simulink model "Teleoperation"  (R2020a)
settings: Solver=VariableStepAuto  StartTime=0.0  StopTime=inf  RelTol=1e-3
undefined symbols (not defined in the file or in its folder): currentCFG_Cognata_Amp_Tobi_split_UB, UB
libraries: robotlib x7, gtecHighspeedLib x2, TobiiEyeTrackerLib x1, gUSBamplib x1
settings Model: Creator=LAB-ORENMUZ  LastModifiedBy=LAB-OREN3
settings DataIOCC: ReturnWorkspaceOutputs=off
settings DebuggingCC: ArithmeticOperatorsInVariantConditions=warning
settings SFSimCC: SimUseLocalCustomCode=off  CustomCodeUndefinedFunction=UseInterfaceOnly
settings RTWCC: RTWUseLocalCustomCode=off
settings CodeAppCC: StateflowObjectComments=on

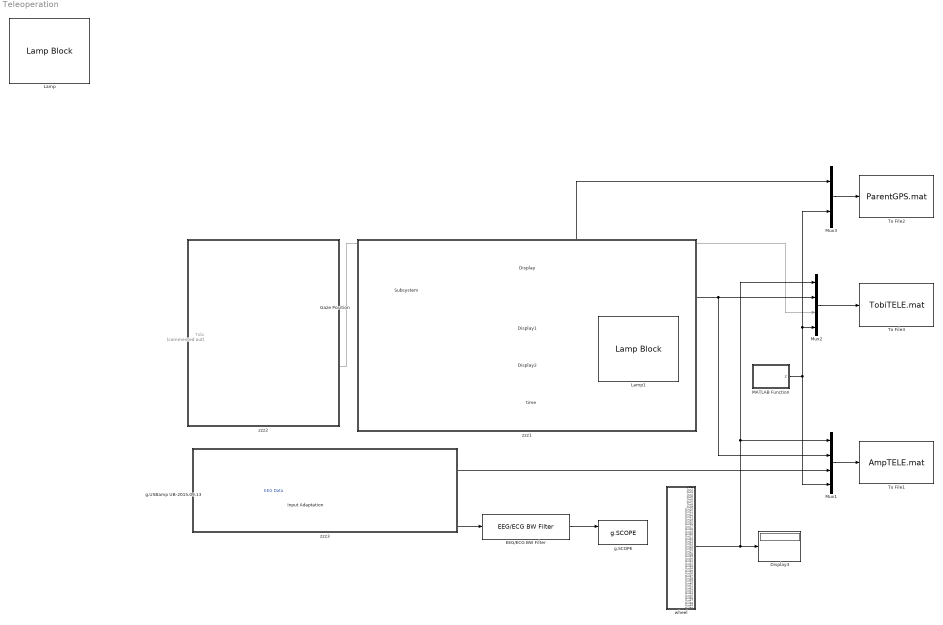
== system Teleoperation ==
  Display{,1..3} (4 alike) : Display
  EEG/ECG BW Filter : gtecHighspeedLib/EEG//ECG BW Filter  Order=6  LowerFreq=0.1  UpperFreq=30  SampFreq=512
      settings: SourceProductName=g.HIsys Library
  Gaze Position : Display
  Input Adaptation : Subsystem
  Lamp : LampBlock
  Lamp1 : LampBlock
  MATLAB Function : MATLAB Function  TreatAsAtomicUnit=on
  Mux1 : Mux
  Mux2 : Mux
  Mux3 : Mux  Inputs=2
  Subsystem : Subsystem
  To File1 : ToFile  Filename=AmpTELE.mat  MatrixName=AmpdataTELE
  To File2 : ToFile  Filename=ParentGPS.mat  MatrixName=Parent
  To File3 : ToFile  Filename=TobiTELE.mat  MatrixName=TobidataTELE
  Tobi : Subsystem  Commented=on
  g.SCOPE : gtecHighspeedLib/g.SCOPE
      settings: SourceProductName=g.HIsys Library
  g.USBamp UB-2015.09.13 : gUSBamplib/g.USBamp  cfg=currentCFG_Cognata_Amp_Tobi_split_UB-2015.09.13.cfg  snr=UB-2015.09.13
      settings: SourceProductName=g.USBamp
  time : Display
  wheel : Subsystem
  zzz1 : Subsystem  TreatAsAtomicUnit=on
      settings: OpenFcn=% no-op
      mask Display: disp('')
  zzz2 : Subsystem  TreatAsAtomicUnit=on
      settings: OpenFcn=% no-op
      mask Display: disp('')
  zzz3 : Subsystem  TreatAsAtomicUnit=on
      settings: OpenFcn=% no-op
      mask Display: disp('')
  wires:
  Subsystem/1(Out1) -> Display/1
  Subsystem/3(Out3) -> Display1/1
  Subsystem/4(Out4) -> Display2/1
  Tobi/2(Sum) -> Mux2/3
  Mux2/1 -> To File3/1
  EEG/ECG BW Filter/1 -> g.SCOPE/1
  Input Adaptation/1(Out) -> Mux1/3, EEG/ECG BW Filter/1
  Tobi/1(Gaze Pos) -> Gaze Position/1
  Subsystem/2(Out2) -> Mux1/2, Mux2/2, Mux3/1
  g.USBamp UB-2015.09.13/1 -> Input Adaptation/1(In)  "EEG Data"
  MATLAB Function/1(z) -> Mux1/4, Mux3/2, Mux2/4
  wheel/25(Out25) -> Mux2/1, Mux1/1, Display3/1
  Mux1/1 -> To File1/1
  Subsystem/5(Out5) -> time/1
  Mux3/1 -> To File2/1

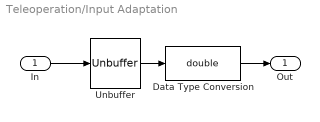
== system Teleoperation/Input Adaptation ==
  In : Inport
  Data Type Conversion : DataTypeConversion  OutDataTypeStr=double
  Unbuffer : Unbuffer
  Out : Outport
  wires:
  In/1 -> Unbuffer/1
  Unbuffer/1 -> Data Type Conversion/1
  Data Type Conversion/1 -> Out/1

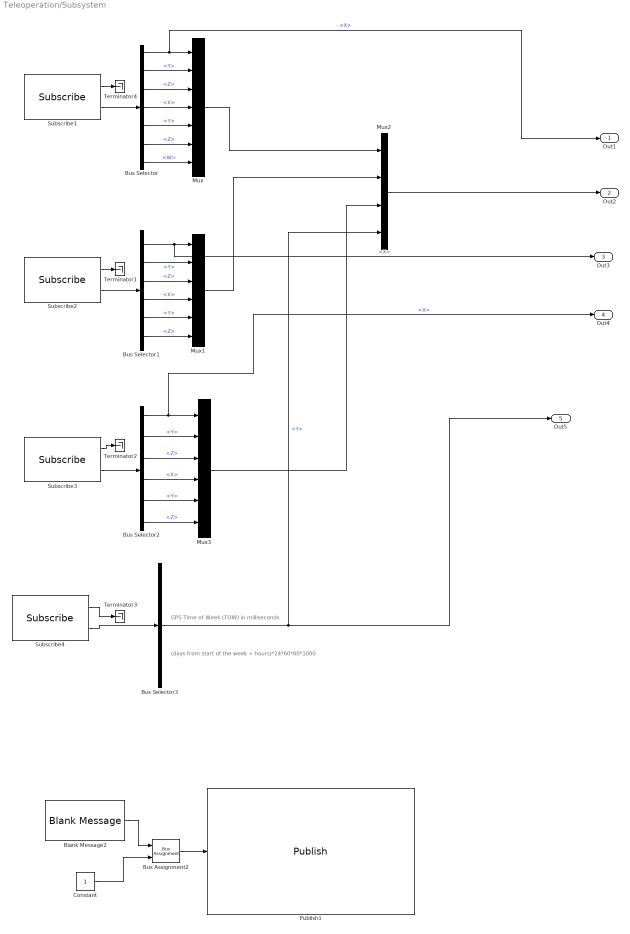
== system Teleoperation/Subsystem ==
  note: GPS Time of Week (TOW) in milliseconds
  note: (days from start of the week + hours)*24*60*60*1000
  Blank Message2 : robotlib/Blank Message  messageClass=Message  entityType=std_msgs/Float64  messageType=std_msgs/Float64  SampleTime=-1
  Bus Assignment2 : BusAssignment  AssignedSignals=Data
  Bus Selector : BusSelector  OutputSignals=Pose.Position.X,Pose.Position.Y,Pose.Position.Z,Pose.Orientation.X,Pose.Orientation.Y,Pose.Orientation.Z,Pose.Orientation.W
  Bus Selector1 : BusSelector  OutputSignals=Twist.Linear.X,Twist.Linear.Y,Twist.Linear.Z,Twist.Angular.X,Twist.Angular.Y,Twist.Angular.Z
  Bus Selector2 : BusSelector  OutputSignals=Twist.Linear.X,Twist.Linear.Y,Twist.Linear.Z,Twist.Angular.X,Twist.Angular.Y,Twist.Angular.Z
  Bus Selector3 : BusSelector  OutputSignals=Twist.Angular.Y
  Constant : Constant
  Mux : Mux  Inputs=7
      settings: DisplayOption=signals
  Mux1 : Mux  Inputs=6
      settings: DisplayOption=signals
  Mux2 : Mux
  Mux3 : Mux  Inputs=6
      settings: DisplayOption=signals
  Publish1 : robotlib/Publish  topicSource=Specify your own  topic=/Record_Flag  messageType=std_msgs/Float64  messageQueueLength=1
  Subscribe1 : robotlib/Subscribe  topicSource=Specify your own  topic=/gnss_pose  messageType=geometry_msgs/PoseStamped  sampleTime=-1  messageQueueLength=10
  Subscribe2 : robotlib/Subscribe  topicSource=Specify your own  topic=/gnss_velocity  messageType=geometry_msgs/TwistStamped  sampleTime=-1  messageQueueLength=10
  Subscribe3 : robotlib/Subscribe  topicSource=Specify your own  topic=/gnss_acceleration  messageType=geometry_msgs/TwistStamped  sampleTime=-1  messageQueueLength=10
  Subscribe4 : robotlib/Subscribe  topicSource=Specify your own  topic=/gps_time  messageType=geometry_msgs/TwistStamped  sampleTime=-1  messageQueueLength=10
  Terminator{1..4} (4 alike) : Terminator
  Out1 : Outport
  Out2 : Outport  Port=2
  Out3 : Outport  Port=3
  Out4 : Outport  Port=4
  Out5 : Outport  Port=5
  wires:
  Bus Selector1/3 -> Mux1/3  "<Z>"
  Mux3/1 -> Mux2/3
  Bus Selector2/3 -> Mux3/3  "<Z>"
  Bus Selector2/6 -> Mux3/6  "<Z>"
  Bus Selector1/4 -> Mux1/4  "<X>"
  Bus Selector/7 -> Mux/7  "<W>"
  Subscribe1/2 -> Bus Selector/1
  Bus Selector/6 -> Mux/6  "<Z>"
  Bus Selector2/2 -> Mux3/2  "<Y>"
  Bus Selector/4 -> Mux/4  "<X>"
  Subscribe2/2 -> Bus Selector1/1
  Bus Selector/3 -> Mux/3  "<Z>"
  Mux2/1 -> Out2/1
  Bus Selector/2 -> Mux/2  "<Y>"
  Subscribe1/1 -> Terminator4/1
  Bus Selector2/4 -> Mux3/4  "<X>"
  Bus Selector/5 -> Mux/5  "<Y>"
  Bus Selector1/2 -> Mux1/2  "<Y>"
  Subscribe3/2 -> Bus Selector2/1
  Bus Selector/1 -> Out1/1, Mux/1  "<X>"
  Bus Selector1/5 -> Mux1/5  "<Y>"
  Mux1/1 -> Mux2/2
  Subscribe3/1 -> Terminator2/1
  Bus Selector1/6 -> Mux1/6  "<Z>"
  Bus Selector2/5 -> Mux3/5  "<Y>"
  Subscribe2/1 -> Terminator1/1
  Mux/1 -> Mux2/1
  Bus Selector2/1 -> Out4/1, Mux3/1  "<X>"
  Bus Selector1/1 -> Out3/1, Mux1/1  "<X>"
  Subscribe4/1 -> Terminator3/1
  Subscribe4/2 -> Bus Selector3/1
  Bus Selector3/1 -> Out5/1, Mux2/4  "<Y>"
  Blank Message2/1 -> Bus Assignment2/1
  Constant/1 -> Bus Assignment2/2
  Bus Assignment2/1 -> Publish1/1

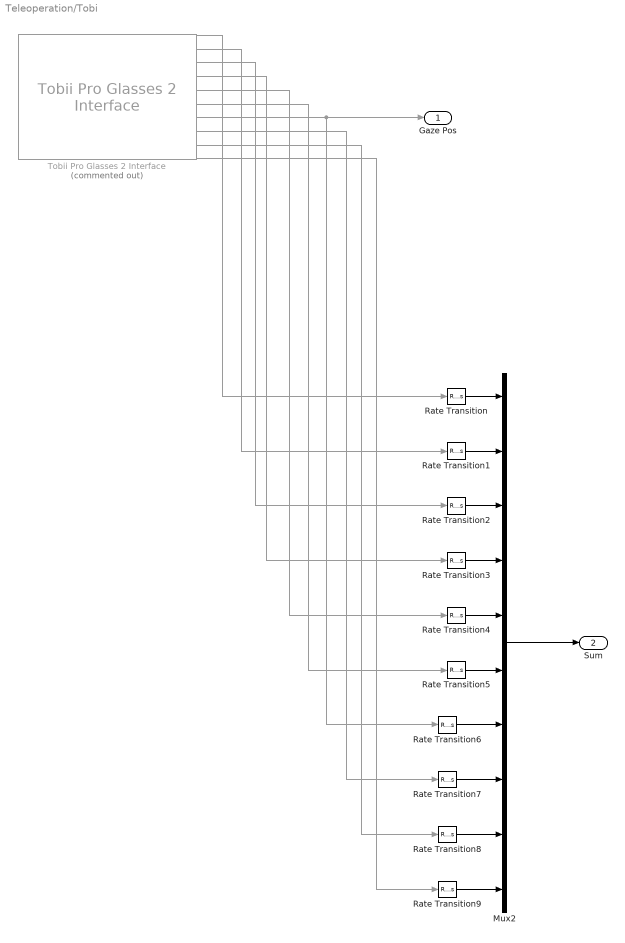
== system Teleoperation/Tobi ==
  Mux2 : Mux  Inputs=10
  Rate Transition{,1..9} (10 alike) : RateTransition  Deterministic=off  OutPortSampleTimeOpt=Inherit
  Tobii Pro Glasses 2 Interface : TobiiEyeTrackerLib/Tobii Pro Glasses 2 Interface  Commented=on  Key=0  pc_right=off  pc_left=off  pd_right=off  pd_left=off  gd_right=off  gd_left=off  gp=on  gp3=off  gy=off  ac=off
      settings: SourceProductName=g.EYEtracking Interface (Tobii Pro Glasses 2)
  Gaze Pos : Outport
  Sum : Outport  Port=2
  wires:
  Rate Transition1/1 -> Mux2/2
  Rate Transition9/1 -> Mux2/10
  Rate Transition6/1 -> Mux2/7
  Rate Transition7/1 -> Mux2/8
  Rate Transition8/1 -> Mux2/9
  Rate Transition/1 -> Mux2/1
  Rate Transition3/1 -> Mux2/4
  Rate Transition5/1 -> Mux2/6
  Rate Transition4/1 -> Mux2/5
  Mux2/1 -> Sum/1
  Rate Transition2/1 -> Mux2/3
  Tobii Pro Glasses 2 Interface/8 -> Rate Transition7/1
  Tobii Pro Glasses 2 Interface/2 -> Rate Transition1/1
  Tobii Pro Glasses 2 Interface/10 -> Rate Transition9/1
  Tobii Pro Glasses 2 Interface/9 -> Rate Transition8/1
  Tobii Pro Glasses 2 Interface/4 -> Rate Transition3/1
  Tobii Pro Glasses 2 Interface/7 -> Gaze Pos/1, Rate Transition6/1
  Tobii Pro Glasses 2 Interface/6 -> Rate Transition5/1
  Tobii Pro Glasses 2 Interface/1 -> Rate Transition/1
  Tobii Pro Glasses 2 Interface/3 -> Rate Transition2/1
  Tobii Pro Glasses 2 Interface/5 -> Rate Transition4/1

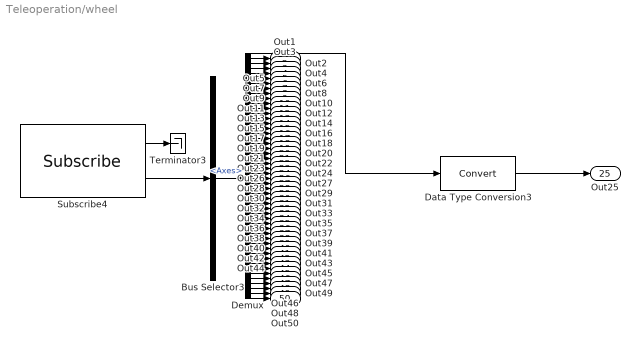
== system Teleoperation/wheel ==
  Bus Selector3 : BusSelector  OutputSignals=Axes
  Data Type Conversion3 : DataTypeConversion
  Demux : Demux  Outputs=50
  Subscribe4 : robotlib/Subscribe  topicSource=Specify your own  topic=/joy  messageType=sensor_msgs/Joy  sampleTime=-1  messageQueueLength=10
  Terminator3 : Terminator
  Out1 : Outport
  Out2 : Outport  Port=2
  Out3 : Outport  Port=3
  Out4 : Outport  Port=4
  Out5 : Outport  Port=5
  Out6 : Outport  Port=6
  Out7 : Outport  Port=7
  Out8 : Outport  Port=8
  Out9 : Outport  Port=9
  Out10 : Outport  Port=10
  Out11 : Outport  Port=11
  Out12 : Outport  Port=12
  Out13 : Outport  Port=13
  Out14 : Outport  Port=14
  Out15 : Outport  Port=15
  Out16 : Outport  Port=16
  Out17 : Outport  Port=17
  Out18 : Outport  Port=18
  Out19 : Outport  Port=19
  Out20 : Outport  Port=20
  Out21 : Outport  Port=21
  Out22 : Outport  Port=22
  Out23 : Outport  Port=23
  Out24 : Outport  Port=24
  Out25 : Outport  Port=25
  Out26 : Outport  Port=26
  Out27 : Outport  Port=27
  Out28 : Outport  Port=28
  Out29 : Outport  Port=29
  Out30 : Outport  Port=30
  Out31 : Outport  Port=31
  Out32 : Outport  Port=32
  Out33 : Outport  Port=33
  Out34 : Outport  Port=34
  Out35 : Outport  Port=35
  Out36 : Outport  Port=36
  Out37 : Outport  Port=37
  Out38 : Outport  Port=38
  Out39 : Outport  Port=39
  Out40 : Outport  Port=40
  Out41 : Outport  Port=41
  Out42 : Outport  Port=42
  Out43 : Outport  Port=43
  Out44 : Outport  Port=44
  Out45 : Outport  Port=45
  Out46 : Outport  Port=46
  Out47 : Outport  Port=47
  Out48 : Outport  Port=48
  Out49 : Outport  Port=49
  Out50 : Outport  Port=50
  wires:
  Demux/2 -> Out1/1
  Demux/3 -> Out2/1
  Demux/4 -> Out3/1
  Demux/5 -> Out4/1
  Demux/6 -> Out5/1
  Demux/7 -> Out6/1
  Demux/8 -> Out7/1
  Demux/10 -> Out9/1
  Demux/9 -> Out8/1
  Demux/11 -> Out10/1
  Demux/13 -> Out12/1
  Demux/12 -> Out11/1
  Demux/15 -> Out14/1
  Demux/31 -> Out31/1
  Demux/19 -> Out18/1
  Demux/30 -> Out30/1
  Demux/16 -> Out15/1
  Demux/32 -> Out32/1
  Demux/33 -> Out33/1
  Demux/34 -> Out34/1
  Demux/14 -> Out13/1
  Demux/20 -> Out19/1
  Demux/17 -> Out16/1
  Demux/22 -> Out21/1
  Demux/23 -> Out22/1
  Demux/26 -> Out26/1
  Demux/24 -> Out23/1
  Demux/21 -> Out20/1
  Demux/27 -> Out27/1
  Demux/28 -> Out28/1
  Demux/18 -> Out17/1
  Demux/25 -> Out24/1
  Demux/29 -> Out29/1
  Demux/37 -> Out37/1
  Demux/39 -> Out39/1
  Demux/36 -> Out36/1
  Demux/38 -> Out38/1
  Demux/45 -> Out45/1
  Demux/41 -> Out41/1
  Demux/35 -> Out35/1
  Demux/44 -> Out44/1
  Demux/40 -> Out40/1
  Demux/43 -> Out43/1
  Demux/42 -> Out42/1
  Demux/46 -> Out46/1
  Bus Selector3/1 -> Demux/1  "<Axes>"
  Data Type Conversion3/1 -> Out25/1
  Subscribe4/2 -> Bus Selector3/1
  Subscribe4/1 -> Terminator3/1
  Demux/1 -> Data Type Conversion3/1
  Demux/48 -> Out48/1
  Demux/50 -> Out50/1
  Demux/49 -> Out49/1
  Demux/47 -> Out47/1

== system Teleoperation/zzz1 ==

== system Teleoperation/zzz2 ==

== system Teleoperation/zzz3 ==

== matlab function Teleoperation/MATLAB Function ==
  data: z output
function z = fcn()
eml.extrinsic('clock'); 
t = [0,0,0,0,0,0];
t = clock;
k = t(1,4:6);
z = k';
end
